simulink model "Practica2PID_224"  (R2014b)
settings: Solver=ode45  StartTime=0.0  StopTime=1000  RelTol=1e-3
libraries: simulink x4
settings Model: Creator=usuario_local  LastModifiedBy=usuario_local

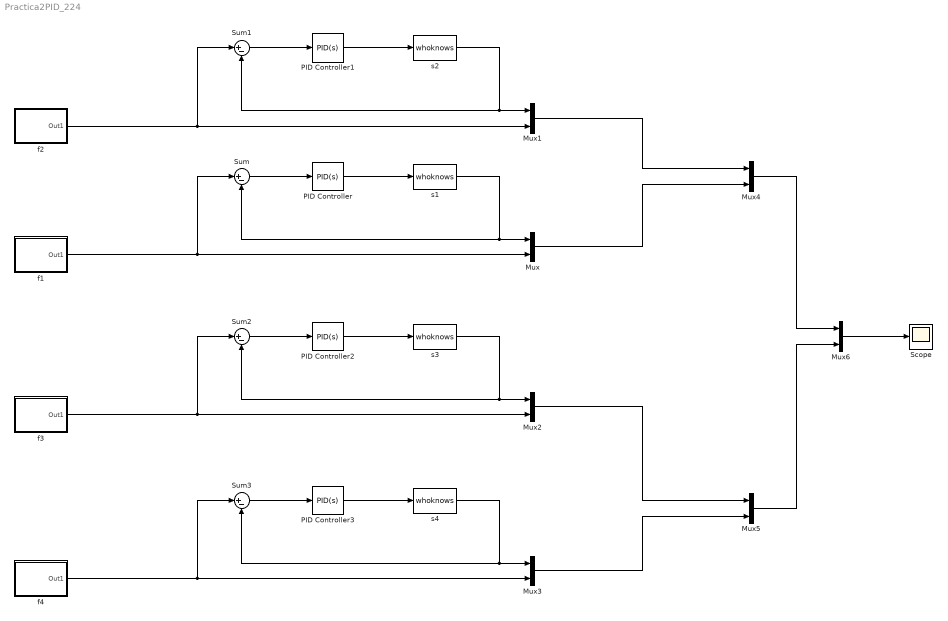
== system Practica2PID_224 ==
  Mux{,1..6} (7 alike) : Mux  Inputs=2
  PID Controller{,1..3} (4 alike) : simulink/Continuous/PID Controller  Controller=PID  TimeDomain=Continuous-time  SampleTime=-1  IntegratorMethod=Forward Euler  FilterMethod=Forward Euler  Form=Parallel  P=0.6 * 0.201  I=(0.6 * 0.201) / (11.5 / 2)  D=(0.6 * 0.201) * (11.5 / 8)  N=100  InitialConditionSource=internal  InitialConditionForIntegrator=0  InitialConditionForFilter=0  ExternalReset=none  LimitOutput=off  UpperSaturationLimit=inf  LowerSaturationLimit=-inf  LinearizeAsGain=on  AntiWindupMode=none  Kb=1  TrackingMode=off  Kt=1  PParamMin=[]  PParamMax=[]  IParamMin=[]  IParamMax=[]  DParamMin=[]  DParamMax=[]  NParamMin=[]  NParamMax=[]  KbParamMin=[]  KbParamMax=[]  KtParamMin=[]  KtParamMax=[]  POutMin=[]  POutMax=[]  IOutMin=[]  IOutMax=[]  DOutMin=[]  DOutMax=[]  NOutMin=[]  NOutMax=[]  KbOutMin=[]  KbOutMax=[]  KtOutMin=[]  KtOutMax=[]  IntegratorOutMin=[]  IntegratorOutMax=[]  FilterOutMin=[]  FilterOutMax=[]  SumOutMin=[]  SumOutMax=[]  SumI1OutMin=[]  SumI1OutMax=[]  SumI2OutMin=[]  SumI2OutMax=[]  SumI3OutMin=[]  SumI3OutMax=[]  SumDOutMin=[]  SumDOutMax=[]  SaturationOutMin=[]  SaturationOutMax=[]  IntegratorContinuousStateAttributes=''  IntegratorStateMustResolveToSignalObject=off  IntegratorRTWStateStorageClass=Auto  FilterContinuousStateAttributes=''  FilterStateMustResolveToSignalObject=off  FilterRTWStateStorageClass=Auto  DifferentiatorICPrevScaledInput=0  DifferentiatorOutMin=[]  DifferentiatorOutMax=[]  UseFilter=on
  Scope : Scope
      settings: YMin=-2  YMax=1
  Sum{,1..3} (4 alike) : Sum  Inputs=|+-
  f1 : Subsystem  mask{S=2, L=0, T=100}
      mask prompts: S "Limite Superior"; L "Limite Inferior"; T "Periodo de cambio"
      mask Display: disp('Ent. Variable')
  f2 : Subsystem  mask{S=1, L=0, T=100}
      mask prompts: S "Limite Superior"; L "Limite Inferior"; T "Periodo de cambio"
      mask Display: disp('Ent. Variable')
  f3 : Subsystem  mask{S=0, L=-1, T=100}
      mask prompts: S "Limite Superior"; L "Limite Inferior"; T "Periodo de cambio"
      mask Display: disp('Ent. Variable')
  f4 : Subsystem  mask{S=0, L=-2, T=100}
      mask prompts: S "Limite Superior"; L "Limite Inferior"; T "Periodo de cambio"
      mask Display: disp('Ent. Variable')
  s1 : M-S-Function  FunctionName=whoknows  Parameters=L, P1, P2, T, R  mask{L=6, P1=0, P2=3, T=2, R=0}
      mask prompts: L "Laboratorio"; P1 "Primer digito del Puesto"; P2 "Segundo digito del Puesto"; T "Tipo de Planta"; R "Ruido"
      mask Display: disp('Sistema')
  s2 : M-S-Function  FunctionName=whoknows  Parameters=L, P1, P2, T, R  mask{L=6, P1=0, P2=3, T=2, R=0}
      mask prompts: L "Laboratorio"; P1 "Primer digito del Puesto"; P2 "Segundo digito del Puesto"; T "Tipo de Planta"; R "Ruido"
      mask Display: disp('Sistema')
  s3 : M-S-Function  FunctionName=whoknows  Parameters=L, P1, P2, T, R  mask{L=6, P1=0, P2=3, T=2, R=0}
      mask prompts: L "Laboratorio"; P1 "Primer digito del Puesto"; P2 "Segundo digito del Puesto"; T "Tipo de Planta"; R "Ruido"
      mask Display: disp('Sistema')
  s4 : M-S-Function  FunctionName=whoknows  Parameters=L, P1, P2, T, R  mask{L=6, P1=0, P2=3, T=2, R=0}
      mask prompts: L "Laboratorio"; P1 "Primer digito del Puesto"; P2 "Segundo digito del Puesto"; T "Tipo de Planta"; R "Ruido"
      mask Display: disp('Sistema')
  wires:
  PID Controller/1 -> s1/1
  Sum/1 -> PID Controller/1
  s1/1 -> Sum/2, Mux/1
  f1/1(Out1) -> Sum/1, Mux/2
  Mux/1 -> Mux4/2
  PID Controller1/1 -> s2/1
  Sum1/1 -> PID Controller1/1
  s2/1 -> Sum1/2, Mux1/1
  f2/1(Out1) -> Sum1/1, Mux1/2
  Mux1/1 -> Mux4/1
  PID Controller2/1 -> s3/1
  Sum2/1 -> PID Controller2/1
  s3/1 -> Sum2/2, Mux2/1
  f3/1(Out1) -> Sum2/1, Mux2/2
  Mux2/1 -> Mux5/1
  PID Controller3/1 -> s4/1
  Sum3/1 -> PID Controller3/1
  s4/1 -> Sum3/2, Mux3/1
  f4/1(Out1) -> Sum3/1, Mux3/2
  Mux3/1 -> Mux5/2
  Mux6/1 -> Scope/1
  Mux4/1 -> Mux6/1
  Mux5/1 -> Mux6/2

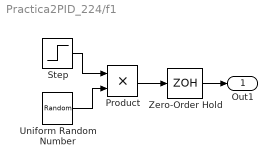
== system Practica2PID_224/f1 ==
  Product : Product  RndMeth=Zero
  Step : Step  Time=0  SampleTime=0
  Uniform Random Number : UniformRandomNumber  Minimum=L  Maximum=S  SampleTime=0
  Zero-Order Hold : ZeroOrderHold  SampleTime=T
  Out1 : Outport
  wires:
  Zero-Order Hold/1 -> Out1/1
  Product/1 -> Zero-Order Hold/1
  Uniform Random Number/1 -> Product/2
  Step/1 -> Product/1

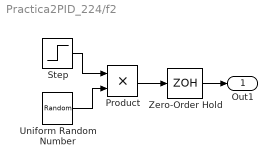
== system Practica2PID_224/f2 ==
  Product : Product  RndMeth=Zero
  Step : Step  Time=0  SampleTime=0
  Uniform Random Number : UniformRandomNumber  Minimum=L  Maximum=S  SampleTime=0
  Zero-Order Hold : ZeroOrderHold  SampleTime=T
  Out1 : Outport
  wires:
  Zero-Order Hold/1 -> Out1/1
  Product/1 -> Zero-Order Hold/1
  Uniform Random Number/1 -> Product/2
  Step/1 -> Product/1

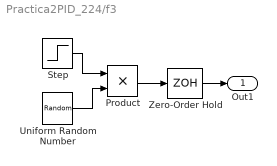
== system Practica2PID_224/f3 ==
  Product : Product  RndMeth=Zero
  Step : Step  Time=0  SampleTime=0
  Uniform Random Number : UniformRandomNumber  Minimum=L  Maximum=S  SampleTime=0
  Zero-Order Hold : ZeroOrderHold  SampleTime=T
  Out1 : Outport
  wires:
  Zero-Order Hold/1 -> Out1/1
  Product/1 -> Zero-Order Hold/1
  Uniform Random Number/1 -> Product/2
  Step/1 -> Product/1

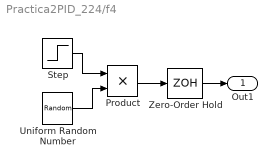
== system Practica2PID_224/f4 ==
  Product : Product  RndMeth=Zero
  Step : Step  Time=0  SampleTime=0
  Uniform Random Number : UniformRandomNumber  Minimum=L  Maximum=S  SampleTime=0
  Zero-Order Hold : ZeroOrderHold  SampleTime=T
  Out1 : Outport
  wires:
  Zero-Order Hold/1 -> Out1/1
  Product/1 -> Zero-Order Hold/1
  Uniform Random Number/1 -> Product/2
  Step/1 -> Product/1
